simulink model "LW_ctrl_241029_1"  (R2024b)
settings: Solver=ode4  StartTime=0.0  StopTime=inf  FixedStep=0.005  RelTol=1e-3  EnableMultiTasking=on
StartFcn:
  | %timestart = cputime;
StopFcn:
  | %dt = cputime - timestart
undefined symbols (not defined in the file or in its folder): AttCtrl_cycle, ControlMode, DEG2RAD, Earth, FlightMode, LW_ACRO_P_MAX, LW_ACRO_R_MAX, LW_ACRO_Y_MAX, LW_AERO_C0, LW_AERO_C1, LW_AERO_Y0, LW_ANGLE, LW_DMZ0, LW_DMZ_MIN, LW_LAT_CIRCLE, LW_MAN_PITCH_MAX, LW_MAN_ROLL_MAX, LW_MASS, LW_OB_CIRCLE_R, LW_OB_CIRCLE_V, LW_OB_CIRCLE_W, LW_OB_TYPE, LW_REX_YAW, LW_SERVOL_MAX, LW_SERVOR_MAX, LW_TEST_DTXY, LW_TEST_DTZ, LW_THR_HOVER, LW_WZ_MAX, LW_X_ACCEL_MAX, LW_X_ACCEL_MIN, LW_X_FF, LW_X_JERK_MAX, LW_X_P, LW_X_VEL_MAX, LW_Y_ACCEL_MAX, LW_Y_ACCEL_MIN, LW_Y_FF, LW_Y_JERK_MAX, LW_Y_P, LW_Y_VEL_MAX, LW_YAW_KAD, LW_YAW_KAP, LW_Z_ACCEL_LOW, LW_Z_ACCEL_UP, LW_Z_FF, LW_Z_JERK_MAX, LW_Z_P, LW_Z_VEL_MAX_UP, Map_xoffset, Map_yoffset, Map_zoffset, MAX_wdotx, MAX_wdoty, MAX_wdotz, Mixer_cycle, ModelParam_AccelMax, ModelParam_DelayAtt, ModelParam_DelayOmega, ModelParam_DelayPos ... (+59)
libraries: pixhawk_slib_uORB_RW x15, simulink x7, slpidlib x6, dspfdesign x6, dspstat3 x5, aerolibnav x4, pixhawk_slib_sensors_actuators x3, aerolibtransform2 x3, etargetslib x2, pixhawk_slib_rfly x1, aerolibatmos2 x1, slrealtimeiplib x1
(part 5 of 6)

== matlab function LW_ctrl_241029_1/Controller/PID_Controller/PID_Controller/local_pos_ref_selector/position control ==
  data: manual_vel_ref input; manual_rates_ref input; offboard_ref input Bus: offboard_bus; timestamp input; vehicle_pos input; vehicle_vel input; delta_xy input size=2; xy_reset_counter input size=1; delta_z input size=1; z_reset_counter input size=1; delta_vxy input size=2; vxy_reset_counter input size=1; delta_vz input size=1; vz_reset_counter input size=1; delta_heading input size=1; heading_reset_counter input size=1; q input; wb input; states_flag input; dm_est input; ctrl_mode input; pos_ref output single; vd_lim output single; flight_mode input; arm input; yaw_ref output; wbz_ref output; man_acc_ff output; LW_WZ_MAX parameter; LW_X_P parameter; LW_Y_P parameter; LW_Z_P parameter; LW_LAT_CIRCLE parameter; LW_X_VEL_MAX parameter; LW_Z_VEL_MAX_UP parameter; LW_X_FF parameter size=1; LW_Y_FF parameter size=1; LW_Z_FF parameter size=1; LW_Y_ACCEL_MAX parameter; LW_REX_YAW parameter; LW_X_JERK_MAX parameter; LW_Y_JERK_MAX parameter; LW_Z_JERK_MAX parameter; LW_DMZ0 parameter; LW_DMZ_MIN parameter; LW_YAW_KAP parameter; LW_YAW_KAD parameter
function [pos_ref, vd_lim, yaw_ref, wbz_ref, man_acc_ff] = fcn(manual_vel_ref, manual_rates_ref, offboard_ref, ...
    timestamp, vehicle_pos, vehicle_vel, delta_xy, xy_reset_counter, delta_z, z_reset_counter,delta_vxy, vxy_reset_counter,delta_vz, vz_reset_counter,delta_heading, heading_reset_counter, q, wb, states_flag, dm_est, ctrl_mode, flight_mode, arm, ...
    LW_WZ_MAX, LW_X_P, LW_Y_P, LW_Z_P, LW_LAT_CIRCLE, LW_X_VEL_MAX, LW_Z_VEL_MAX_UP, LW_X_FF, LW_Y_FF, LW_Z_FF, LW_Y_ACCEL_MAX, LW_REX_YAW, LW_X_JERK_MAX, LW_Y_JERK_MAX, LW_Z_JERK_MAX,...
    LW_DMZ0, LW_DMZ_MIN, LW_YAW_KAP, LW_YAW_KAD)
%Function description:
%  Mode switch implementation.
%Input:
%  mode
%  manual_vel_ref：航向坐标系下的期望速度
%  vel_ref: The desired velocity specified by the remote control
%  x, y, z: current position
%  vx, vy,vz: current velocity
%Output:
%  pos_ref, vd_lim: desired velocity and position in NED

lw_acc_xy_max = LW_Y_ACCEL_MAX; %水平方向最大减速加速度
lw_acc_z_max = single(3.0);
if notInfNan(q)
    yaw = my_quat2yaw(q,'ZYX');%强制旋转次序，很有必要
else
    yaw = single(0);
end

%% persistent data define
persistent timestamp_last
if isempty(timestamp_last)
    timestamp_last = timestamp;
    dt = single(0.02);
else
    dt = single((timestamp - timestamp_last)*1e-6);
end
if dt > 0.2
    dt = single(0.2);
elseif dt < 0.001
    dt = single(0.001);
end
timestamp_last = timestamp;

persistent pos_x1 pos_y1 pos_z1
if isempty(pos_x1) || isempty(pos_y1) || isempty(pos_z1)
    if notInfNan(vehicle_pos)
        pos_x1 = vehicle_pos(1);
        pos_y1 = vehicle_pos(2);
        pos_z1 = vehicle_pos(3);
    else
        pos_x1 = single(0);
        pos_y1 = single(0);
        pos_z1 = single(0);
    end
end
persistent hold_xy_flag  hold_z_flag;
if isempty(hold_xy_flag) || isempty(hold_z_flag)
    hold_xy_flag = false;
    hold_z_flag = false;
end
persistent yaw_d_
if isempty(yaw_d_)
    if notInfNan(yaw)
        yaw_d_ = yaw;
    else
        yaw_d_ = single(0);
    end
end
persistent hold_xy_timestamp  hold_z_timestamp hold_vxy hold_pxy hold_vz hold_pz;
if isempty(hold_xy_timestamp) || isempty(hold_z_timestamp)
    hold_xy_timestamp = timestamp;
    hold_z_timestamp = timestamp;
end
if isempty(hold_vxy)
    hold_vxy = vehicle_vel(1:2);
end
if isempty(hold_pxy)
    hold_pxy = vehicle_pos(1:2);
end
if isempty(hold_pz)
    hold_pz = vehicle_pos(3);
end
if isempty(hold_vz)
    hold_vz = vehicle_vel(3);
end

persistent xy_reset_counter_ z_reset_counter_ vxy_reset_counter_ vz_reset_counter_ heading_reset_counter_
if isempty(heading_reset_counter_) || isempty(xy_reset_counter_) || isempty(z_reset_counter_) ...
        || isempty(vxy_reset_counter_) || isempty(vz_reset_counter_)
    xy_reset_counter_ = xy_reset_counter;
    z_reset_counter_ = z_reset_counter;
    vxy_reset_counter_ = vxy_reset_counter;
    vz_reset_counter_ = vz_reset_counter;
    heading_reset_counter_ = heading_reset_counter;
end

man_acc_ff = zeros(3,1,'single');
if notInfNan(flight_mode) && notInfNan(ctrl_mode) && arm == ControlMode.ARM
    %% yaw control
    relaxed_yaw = states_flag(1);
    wbz_ref = single(0);
    if flight_mode == FlightMode.PILOT && notInfNan(manual_rates_ref)...
            && ctrl_mode == ControlMode.POSITION
        if hold_xy_flag && LW_REX_YAW > 0.5 && abs(manual_rates_ref(3)) < 0.01
            Euler = my_quat2eul(q,'ZYX');
            dot_yaw = sin(Euler(1))/cos(Euler(2))*wb(2) + cos(Euler(1))/cos(Euler(2))*wb(3);
            if LW_YAW_KAD > 0.001
                [yaw_d_, dot_yaw_ref] = AdmittanceYaw(dm_est(3), yaw, dot_yaw, dt, LW_DMZ0, LW_DMZ_MIN, LW_YAW_KAP, LW_YAW_KAD, 0);
                wbz_ref = dot_yaw_ref*cos(Euler(1))*cos(Euler(2));
                wbz_ref = single(0);
            else
                roll_min = LW_DMZ_MIN;
                wv_gain = LW_YAW_KAP;
                roll_exceeding_treshold = single(0);
                if Euler(1) > roll_min
                    roll_exceeding_treshold = Euler(1) - roll_min;
                elseif Euler(1) < -roll_min
                    roll_exceeding_treshold = Euler(1) + roll_min;
                end
                yaw_d_ = yaw;
                wbz_ref = wv_gain*roll_exceeding_treshold;
            end
            %             if relaxed_yaw > 0.5
            %                 yaw_d_ = yaw;%悬停状态放宽偏航控制
            %             end
        else
            [~, ~] = AdmittanceYaw(dm_est(3), yaw, single(0), dt, LW_DMZ0, LW_DMZ_MIN, LW_YAW_KAP, LW_YAW_KAD, 1);%reset
            yaw_d_ = yaw_d_ + manual_rates_ref(3) * dt; %前飞状态允许手控偏航
        end
        if my_norm(vehicle_vel(1:2)) > 3 && abs(manual_vel_ref(2)) > 0.1
            yaw_d_ = yaw;
        end
    else
        yaw_d_ = yaw;
        [~, ~] = AdmittanceYaw(dm_est(3), yaw, single(0), dt, LW_DMZ0, LW_DMZ_MIN, LW_YAW_KAP, LW_YAW_KAD, 1); %reset
    end

    if flight_mode == FlightMode.PILOT
        %handle reset
        if heading_reset_counter_ ~= heading_reset_counter && abs(wrap_pi(yaw_d_ - yaw)) > 0.001
            yaw_d_ = yaw_d_ + delta_heading;
        end
        yaw_ref = yaw_d_;
    elseif flight_mode == FlightMode.OFFBOARD
        yaw_ref = my_quat2yaw(offboard_ref.q,'ZYX');%已经经过了reset补偿
    else
        yaw_ref = yaw_d_;
    end

    %限定偏航角的最大角度率
    LW_WZ_MAX_RAD = LW_WZ_MAX * pi / 180;
    %yaw_ref = limit_yaw(yaw_ref, dt, LW_WZ_MAX_RAD, arm);

    Rbe_psi = [ cos(yaw_d_) sin(yaw_d_) 0;
        -sin(yaw_d_) cos(yaw_d_) 0;
        0        0        1];

    %% select reference data
    if flight_mode == FlightMode.PILOT && (notInfNan(vehicle_pos) && notInfNan(vehicle_vel) && notInfNan(manual_vel_ref))
        vehicle_vel_psi = Rbe_psi*vehicle_vel;
        if ctrl_mode == ControlMode.STABILIZED || ctrl_mode == ControlMode.ACRO || ctrl_mode == ControlMode.MANUAL
            pos_x1 = vehicle_pos(1); pos_y1 = vehicle_pos(2); pos_z1 = vehicle_pos(3);
            hold_pxy = vehicle_pos(1:2); hold_pz = vehicle_pos(3);
            hold_vxy = vehicle_vel(1:2); hold_vz = vehicle_vel(3);
            hold_z_flag = false; hold_xy_flag = false;
            hold_xy_timestamp = timestamp; hold_z_timestamp = timestamp;
            vx_d = vehicle_vel_psi(1); vy_d = vehicle_vel_psi(2); vz_d = vehicle_vel_psi(3);
        elseif ctrl_mode == ControlMode.ALTITUDE
            pos_x1 = vehicle_pos(1); pos_y1 = vehicle_pos(2);
            hold_pxy = vehicle_pos(1:2);
            hold_vxy = vehicle_vel(1:2);
            hold_xy_flag = false;
            hold_xy_timestamp = timestamp;
            vx_d = vehicle_vel_psi(1); vy_d = vehicle_vel_psi(2);
            %判断是否需要定高
            if abs(manual_vel_ref(3)) < 0.001 && abs(vehicle_vel(3)) <= 0.8
                want_hold_z = true;
            else
                want_hold_z = false;
                hold_z_flag = false;
                hold_z_timestamp = timestamp;
                hold_vz = vehicle_vel(3);
                hold_pz = vehicle_pos(3);
            end

            if (want_hold_z) && (~hold_z_flag)
                %加入最大加速度限制
                time_to_stop = my_norm(hold_vz)/lw_acc_z_max;
                delta_t = single((timestamp - hold_z_timestamp)*1e-6);
                if delta_t > time_to_stop
                    delta_t = time_to_stop;
                    hold_z_flag = true;
                end
                pos_z1 = hold_pz + hold_vz*delta_t;
            end

            if ~want_hold_z
                pos_z1 = vehicle_pos(3);
                hold_z_flag = false;
            end
            vz_d = manual_vel_ref(3);
        else %position mode
            if abs(manual_vel_ref(1)) < 0.001 && abs(vehicle_vel_psi(1)) <= 0.8 && ...
                    abs(manual_vel_ref(2)) < 0.001 && abs(vehicle_vel_psi(2)) <= 0.8
                want_hold_xy = true;
            else
                want_hold_xy = false; hold_xy_flag = false;
                hold_xy_timestamp = timestamp;
                hold_vxy = vehicle_vel(1:2);
                hold_pxy = vehicle_pos(1:2);
            end
            if abs(manual_vel_ref(3)) < 0.001 && abs(vehicle_vel(3)) <= 0.8
                want_hold_z = true;
            else
                want_hold_z = false;
                hold_z_flag = false;
                hold_z_timestamp = timestamp;
                hold_vz = vehicle_vel(3);
                hold_pz = vehicle_pos(3);
            end

            vx_d = manual_vel_ref(1); vy_d = manual_vel_ref(2);
            vz_d = manual_vel_ref(3);
            %对手动期望速度进行平滑
            %             [vd_smoothed, ~] = TD_3DVector([vx_d;vy_d;vz_d], [lw_acc_xy_max;lw_acc_xy_max;lw_acc_z_max]*1.2, dt);
            %             vx_d = vd_smoothed(1);
            %             vy_d = vd_smoothed(2);
            %             vz_d = vd_smoothed(3);
            %让期望位置保持进入定点那刻的位置
            if (want_hold_xy) && (~hold_xy_flag)
                %加入最大加速度限制
                v0_xy = my_norm(hold_vxy(1:2));
                time_to_stop = v0_xy/lw_acc_xy_max;
                delta_t = single((timestamp - hold_xy_timestamp)*1e-6);
                if delta_t > time_to_stop
                    delta_t = time_to_stop;
                    hold_xy_flag = true;
                end

                pos_x1 = hold_pxy(1) + hold_vxy(1)*delta_t;
                pos_y1 = hold_pxy(2) + hold_vxy(2)*delta_t;

                %                 delta_vxy = v0_xy - lw_acc_xy_max*delta_t;
                %                 delta_pxy = v0_xy*delta_t - 0.5*lw_acc_xy_max*delta_t^2;
                %                 pos_x1 = hold_pxy(1) + delta_pxy*cos(yaw_d_);
                %                 pos_y1 = hold_pxy(2) + delta_pxy*sin(yaw_d_);

                %直接停住
                %                     x1 = vehicle_pos(1); y1 = vehicle_pos(2);
                %                     hold_xy_flag = true;
            end

            % throttle in the middle position, hold the height
            if (want_hold_z) && (~hold_z_flag)
                %加入最大加速度限制
                time_to_stop = my_norm(hold_vz)/lw_acc_z_max;
                delta_t = single((timestamp - hold_xy_timestamp)*1e-6);
                if delta_t > time_to_stop
                    delta_t = time_to_stop;
                    hold_z_flag = true;
                end
                pos_z1 = hold_pz + hold_vz*delta_t;
            end
            %When the RC sticks(CH1, CH2, CH3, CH4) deviate from the middle dead zone range, the position is the current position.
            %The position controller only works with the velocity loop
            if ~want_hold_xy
                pos_x1 = vehicle_pos(1); pos_y1 = vehicle_pos(2);
                hold_xy_flag = false;
            end
            if ~want_hold_z
                pos_z1 = vehicle_pos(3); hold_z_flag = false;
            end

        end
        vel_ref = [vx_d; vy_d; vz_d]; %航向坐标系下的期望速度
        pos_ref = [pos_x1; pos_y1; pos_z1];

        % 状态reset处理
        delta_v = Rbe_psi *[delta_vxy;delta_vz];
        if vxy_reset_counter_ ~= vxy_reset_counter && my_norm(vel_ref(1:2) - vehicle_vel(1:2)) > 0.001
            vel_ref(1:2) = vel_ref(1:2) + delta_v(1:2);
        end
        if vz_reset_counter_ ~= vz_reset_counter && abs(vel_ref(3) - vehicle_vel(3)) > 0.001
            vel_ref(3) = vel_ref(3) +  delta_v(3);
        end
        if xy_reset_counter_ ~= xy_reset_counter && my_norm(pos_ref(1:2) - vehicle_pos(1:2)) > 0.001
            pos_ref(1:2) = pos_ref(1:2) + delta_xy;
            pos_x1 = pos_ref(1);
            pos_y1 = pos_ref(2);
        end
        if z_reset_counter_ ~= z_reset_counter && abs(pos_ref(3) - vehicle_pos(3)) > 0.001
            pos_ref(3) = pos_ref(3) + delta_z;
            pos_z1 = pos_ref(3);
        end
        xy_reset_counter_ = xy_reset_counter;
        z_reset_counter_ = z_reset_counter;
        vxy_reset_counter_ = vxy_reset_counter;
        vz_reset_counter_ = vz_reset_counter;
        heading_reset_counter_ = heading_reset_counter;
        %
        %     elseif flight_mode == FlightMode.AUTO && notInfNan(vehicle_pos) % auto
        %         dubins = auto_ref.dubins;
        %         pos_ref = [vehicle_pos(1 : 2); -non_manual_ref.current.alt];
        %         vel_ref = [non_manual_ref.current.cruising_speed; 0; 0];
        %         x1 = vehicle_pos(1); y1 = vehicle_pos(2); z1 = vehicle_pos(3);
        %         if ctrl_mode == ControlMode.LOITER && (notInfNan(non_manual_ref.current.pos) && notInfNan(non_manual_ref.current.vel))
        %             pos_ref = non_manual_ref.current.pos;
        %             vel_ref = non_manual_ref.current.vel;
        %         end
    elseif flight_mode == FlightMode.OFFBOARD && (notInfNan(vehicle_pos)) % offboard
        if notInfNan(offboard_ref.pos)
            pos_ref = offboard_ref.pos;
        else
            pos_ref = vehicle_pos;
        end
        if notInfNan(offboard_ref.vel)
            vel_ref = offboard_ref.vel;
        else
            vel_ref = zeros(3,1,'single');
        end

        pos_x1 = vehicle_pos(1); pos_y1 = vehicle_pos(2); pos_z1 = vehicle_pos(3);
        hold_pxy = vehicle_pos(1:2); hold_pz = vehicle_pos(3);
        hold_vxy = vehicle_vel(1:2); hold_vz = vehicle_vel(3);
        hold_z_flag = false; hold_xy_flag = false;
        hold_xy_timestamp = timestamp; hold_z_timestamp = timestamp;
    else
        vel_ref = single([0; 0; 0]);
        pos_ref = [pos_x1; pos_y1; pos_z1];
    end


    %% position control
    vel_fb = (pos_ref - vehicle_pos).* [LW_X_P; LW_Y_P; LW_Z_P];
    vd_psi = Rbe_psi *vel_fb + vel_ref; %手控模式下参考速度vel_ref是航向坐标系下的
    if flight_mode == FlightMode.AUTO  %not used, replaced by the L1 in PX4
        if vel_ref(2) < 1e-3
            vd_psi(2) = vel_fb(2);
        else
            %对圆轨迹跟踪，d为半径误差
            vd_psi(2) = single(LW_LAT_CIRCLE * vel_ref(2));
        end
    end

    vd_lim = Rbe_psi'*vd_psi;%将期望速度转换到NED下
    if (flight_mode == FlightMode.PILOT && (ctrl_mode == ControlMode.ALTITUDE || ctrl_mode == ControlMode.POSITION )) ...
            || flight_mode == FlightMode.AUTO
        %z-axis保大小
        vd_psi(3) = constrain(vd_psi(3), -LW_Z_VEL_MAX_UP, LW_Z_VEL_MAX_UP);

        if (flight_mode == FlightMode.PILOT && (ctrl_mode == ControlMode.POSITION )) || flight_mode == FlightMode.AUTO
            %xy-axis保方向
            vd_xy_norm = sqrt(vd_psi(1) * vd_psi(1) + vd_psi(2) * vd_psi(2));
            VEL_MAX_XY = LW_X_VEL_MAX;
            if vd_xy_norm > VEL_MAX_XY
                vd_psi(1 : 2) = vd_psi(1 : 2) * VEL_MAX_XY / vd_xy_norm;
            end
        end
        [vd_psi, man_acc_ff] = TD_3DVector(vd_psi, ([LW_X_JERK_MAX; LW_Y_JERK_MAX; LW_Z_JERK_MAX]), dt);
        man_acc_ff = zeros(3,1,'single');%手动控制加速度前馈
        vd_lim = Rbe_psi'*vd_psi;
    end
    if flight_mode == FlightMode.OFFBOARD
        vel_fb = ((pos_ref - vehicle_pos)).* [LW_X_P; LW_Y_P; LW_Z_P];
        vd_lim = vel_fb + vel_ref.* [LW_X_FF; LW_Y_FF; LW_Z_FF];
    end
else
    if notInfNan(vehicle_pos)
        pos_ref = vehicle_pos;
    else
        pos_ref = single([0; 0; 0]);
    end
    vd_lim = single([0; 0; 0]);
    yaw_ref = yaw;
    wbz_ref = single(0);
    [~, ~] = AdmittanceYaw(dm_est(3), yaw, single(0), dt, LW_DMZ0, LW_DMZ_MIN, LW_YAW_KAP, LW_YAW_KAD, 1); %reset

    pos_x1 = vehicle_pos(1); pos_y1 = vehicle_pos(2); pos_z1 = vehicle_pos(3);
    hold_pxy = vehicle_pos(1:2); hold_pz = vehicle_pos(3);
    hold_vxy = vehicle_vel(1:2); hold_vz = vehicle_vel(3);
    hold_z_flag = false; hold_xy_flag = false;
    hold_xy_timestamp = timestamp; hold_z_timestamp = timestamp;
    yaw_d_ = yaw;

    xy_reset_counter_ = xy_reset_counter;
    z_reset_counter_ = z_reset_counter;
    vxy_reset_counter_ = vxy_reset_counter;
    vz_reset_counter_ = vz_reset_counter;
    heading_reset_counter_ = heading_reset_counter;
end
%yaw_ref = my_quat2yaw(offboard_ref.q,'ZYX');
%yaw_ref = single(45/180*pi);
end

function [yaw_ref, dot_yaw_ref] = AdmittanceYaw(dmz, yaw, dot_yaw, dt, dmz0, dmz_min, k_ap, k_ad, reset)
% 偏航导纳控制
% 误差形式：
% e = yaw_ref - yaw
% k_ap*e + k_ad*dote = dmz
% 输入：
% dmz         - 估计偏航力矩扰动 d_m_est_z
% yaw         - 偏航角 \psi
% dot_yaw     - 偏航导数 \dot{\psi}
% dt          - 采样时间间隔
% 输出：
% yaw_ref     - 期望偏航角
% dot_yaw_ref - 期望偏航角速率
% 参数：
% k_ad        - 调节参数 k_{\text{ad}}
% k_ap        - 调节参数 k_{\text{ap}}


persistent yawerror_last yaw_ref_last
if isempty(yawerror_last) || isempty(yaw_ref_last)
    yawerror_last = single(0);
    yaw_ref_last =  yaw;
end

% k_ap = 1; k_ad = 1.0;
% dmz0 = -0.023;
if reset > 0.5
    yawerror_last = single(0);
    yaw_ref_last =  yaw;
    yaw_ref = yaw;
    dot_yaw_ref = single(0);
else
    dmz = dmz - dmz0;
    if abs(dmz) <= dmz_min
        dmz = single(0);
    end
    dot_yaw_ref = dot_yaw + 1/k_ad*(-k_ap*yawerror_last + dmz);
    yawerror_last = yawerror_last + (dot_yaw_ref - dot_yaw)*dt;
    yaw_ref = yaw + yawerror_last;

    if abs(dmz) <= dmz_min
        yaw_ref = yaw_ref_last;
    else
        yaw_ref_last = yaw_ref;
    end
end

end

function yaw_lim = limit_yaw(yaw_ref, dt, wz_max, arm)
persistent yaw_d_last;
if isempty(yaw_d_last)
    yaw_d_last = single(yaw_ref);
end
yaw_error = yaw_ref - yaw_d_last;
yaw_error = wrap_pi(yaw_error);
yawrate_ref = yaw_error / dt;

if yawrate_ref > wz_max
    yaw_ref = yaw_d_last + wz_max * dt;
elseif yawrate_ref < -wz_max
    yaw_ref = yaw_d_last - wz_max * dt;
end
yaw_lim = wrap_pi(yaw_ref);
if arm == ControlMode.ARM
    yaw_d_last = yaw_lim;
else
    yaw_d_last = yaw_ref;
end
end

function [v1_, v2_] = TD_3DVector(v, r, h)
%v:[3,1]
%r:[3,1]
%h:1
persistent v1 v2
if isempty(v1) || isempty(v2)
    v1 = single([0;0;0]);
    v2 = single([0;0;0]);
end
v = single(v);
r = single(r);
h = single(h);

v1_ = v1;
v2_ = v2;
for i = 1:3
    fv = fhan(v1(i) - v(i), v2(i), r(i),  h);
    v1_(i) = v1(i) + h*v2(i);
    v2_(i) = v2(i) + h*fv;
end

if notInfNan(v1_) && notInfNan(v2_)
    v1 = v1_;
    v2 = v2_;
end
end

function y = fhan(x1, x2, r0, h0)

d = r0*h0^2;
a0 = h0*x2;
y = x1 + a0;
a1 = sqrt(d*(d + 8*abs(y)));
a2 = a0 + sign(y)*(a1 - d)/2;
sy = (sign(y + d) - sign(y - d))/2;%fsg
a = (a0 + y -a2)*sy + a2;
sa = (sign(a + d) - sign(a - d))/2;
y = -r0*(a/d - sign(a))*sa - r0*sign(a);

end

== matlab function LW_ctrl_241029_1/navigator/navigator_manual/nan_inf11 ==
  data: u input; y output
function y = fcn(u)

for i = 1:length(u)
    if isnan(u(i)) || isinf(u(i))
        u(i) = single(0);
    end
end
y = u;

== matlab function LW_ctrl_241029_1/navigator/navigator_manual/nan_inf9 ==
  data: u input; y output
function y = fcn(u)

for i = 1:length(u)
    if isnan(u(i)) || isinf(u(i))
        u(i) = single(0);
    end
end
y = u;

== matlab function LW_ctrl_241029_1/navigator/navigator_manual/pitchrate_deadzone1 ==
  data: u input; y output
function y = fcn(u)
%Function description:
%  set a dead zone with a dead zone size of ±deadZone.
RCMin = single(-1);
RCMax = single(1);
RCMid = ((RCMin + RCMax)/2);
deadZone = 0;
k = 1/(RCMax - RCMid - deadZone);

%dead zone
if(u > RCMid + deadZone)
    y = single((u-RCMid - deadZone)*k);
elseif(u < RCMid - deadZone)
    y = single((u - RCMid + deadZone)*k);
else
    y = single(0);
end
end

== matlab function LW_ctrl_241029_1/Controller/PID_Controller/PID_Controller/altitude control/attrates_ref_selector ==
  data: flight_mode input; arm input; ctrl_mode input; rate_ctrl_integral_reset output
function rate_ctrl_integral_reset = fcn(flight_mode, arm, ctrl_mode)

rate_ctrl_integral_reset = [true; true; true];
if notInfNan(flight_mode) && notInfNan([ctrl_mode, arm])
    if  arm == ControlMode.DISARM || ctrl_mode == ControlMode.MANUAL
        rate_ctrl_integral_reset = [true; true; true];
    else
        rate_ctrl_integral_reset = [false; false; false];
    end
end

end

== matlab function LW_ctrl_241029_1/Controller/PID_Controller/PID_Controller/postion control/nan_inf_mode ==
  data: u input; y output
function y = fcn(u)

for i = 1:length(u)
    if isnan(u(i)) || isinf(u(i))
        u(i) = ControlMode.DISARM;
    end
end
y = u;

== matlab function LW_ctrl_241029_1/Controller/PID_Controller/PID_Controller/postion control/pos_ctrl_integral_reset ==
  data: ctrl_mode input; integral_reset output boolean
function integral_reset = fcn(ctrl_mode)
mode = ctrl_mode(1);
arm = ctrl_mode(2);
if mode == ControlMode.ACRO || mode == ControlMode.STABILIZED || mode == ControlMode.MANUAL || arm == ControlMode.DISARM
    integral_reset = [true true];
elseif mode == ControlMode.ALTITUDE
    integral_reset = [true false];
elseif mode == ControlMode.POSITION
    integral_reset = [false false];
else
    integral_reset = [false false];
end

== matlab function LW_ctrl_241029_1/Controller/PID_Controller/PID_Controller/postion control/pos_ctrl_integral_reset2 ==
  data: v_ned input; v_body output; psi input
function v_body = fcn(v_ned, psi)
    % 构造旋转矩阵
    R = [cos(psi), sin(psi), 0;
         -sin(psi), cos(psi), 0;
         0, 0, 1];

    % 转换速度
    v_body = R * [v_ned(1);v_ned(2);v_ned(3)];
end

== matlab function LW_ctrl_241029_1/Controller/PID_Controller/PID_Controller/postion control/pos_ctrl_integral_reset3 ==
  data: eax input; phi_d output; eay input; theta_d output
function [phi_d,theta_d] = fcn(eax,eay)

g = 9.8;
phi_d = atan(eay/g);
theta_d = -atan(eax/g);

== matlab function LW_ctrl_241029_1/Controller/PID_Controller/PID_Controller/select parameter/MATLAB Function ==
  data: u input; y output
function y = fcn(u)

y = my_quat2eul(u);

== matlab function LW_ctrl_241029_1/Controller/PID_Controller/PID_Controller/altitude control/MATLAB Function ==
  data: f_d input; Mx_d input; My_d input; T1 output; Mz_d input; T2 output; T3 output; T4 output; ModelParam_uavJ parameter
function [T1,T2,T3,T4] = fcn(f_d,Mx_d,My_d,Mz_d,ModelParam_uavJ)


u = ModelParam_uavJ*[Mx_d;My_d;Mz_d];
fM_d = [f_d;u];
Allocation = [0.2500   -1.1765    1.0000   15.0602
    0.2500   -1.1765   -1.0000  -15.0602
    0.2500    1.1765    1.0000  -15.0602
    0.2500    1.1765   -1.0000   15.0602];

T = Allocation*fM_d;
if T(1)<0
    T1 = single(0);
else
    T1 = T(1);
end
if T(2)<0
    T2 = single(0);
else
    T2 = T(2);
end
if T(3)<0
    T3 = single(0);
else
    T3 = T(3);
end
if T(4)<0
    T4 = single(0);
else
    T4 = T(4);
end

== matlab function LW_ctrl_241029_1/Controller/PID_Controller/PID_Controller/altitude control/MATLAB Function1 ==
  data: quat input; euler_d input; psi_err output; phi_err output; theta_err output
function [psi_err,phi_err,theta_err] = fcn(quat,euler_d)

quat_d = my_eul2quat(euler_d);
euler = my_quat2eul(quat);

% quat_d, quat: 1x4, [w x y z]
q_err = quatmultiply(quat_d', quatinv(quat')); 

eul_err = quat2eul(q_err, "ZYX");              
psi_err = 3*wrapToPi(eul_err(1));                
phi_err = 10*(euler_d(1) - euler(1));
theta_err = 10*(euler_d(2) - euler(2));

== matlab function LW_ctrl_241029_1/Controller/PID_Controller/PID_Controller/postion control/pos_ctrl_integral_reset1 ==
  data: v_ned input; psi input; v_body output
function v_body  = fcn(v_ned, psi)
    % 构造旋转矩阵
    R = [cos(psi), sin(psi), 0;
         -sin(psi), cos(psi), 0;
         0, 0, 1];

    % 转换速度
    v_body = R * [v_ned(1);v_ned(2);v_ned(3)];
end

== matlab function LW_ctrl_241029_1/navigator/navigator_manual/rollrate_deadzone1 ==
  data: u input; y output
function y = fcn(u)
%Function description:
%  set a dead zone with a dead zone size of ±deadZone.
RCMin = single(-1);
RCMax = single(1);
RCMid = ((RCMin + RCMax)/2);
deadZone = 0;
k = 1/(RCMax - RCMid - deadZone);

%dead zone
if(u > RCMid + deadZone)
    y = single((u-RCMid - deadZone)*k);
elseif(u < RCMid - deadZone)
    y = single((u - RCMid + deadZone)*k);
else
    y = single(0);
end
end

== matlab function LW_ctrl_241029_1/navigator/navigator_manual/yawrate_deadzone1 ==
  data: u input; y output
function y = fcn(u)
%Function description:
%  set a dead zone with a dead zone size of ±deadZone.
RCMin = single(-1);
RCMax = single(1);
RCMid = ((RCMin + RCMax)/2);
deadZone = 0;
k = 1/(RCMax - RCMid - deadZone);

%dead zone
if(u > RCMid + deadZone)
    y = single((u-RCMid - deadZone)*k);
elseif(u < RCMid - deadZone)
    y = single((u - RCMid + deadZone)*k);
else
    y = single(0);
end
end

== matlab function LW_ctrl_241029_1/rc_receive/manual_ctrl_in/Sim/Simulate ref/commandMapping/command2pwm/man/delta_e_inv ==
  data: u input; y output
function y = fcn(u)
%Function description:
%  set a dead zone with a dead zone size of ±deadZone.
RCMin = single(-1);
RCMax = single(1);
RCMid = ((RCMin + RCMax)/2);
deadZone = 0;
k = 1/(RCMax - RCMid - deadZone);

%dead zone
if(u > RCMid + deadZone)
    y = single(u/k + RCMid + deadZone);
elseif(u < RCMid - deadZone)
     y = single(u/k + RCMid - deadZone);
else
    y = single(0);
end
end

== matlab function LW_ctrl_241029_1/rc_receive/manual_ctrl_in/Sim/Simulate ref/commandMapping/command2pwm/man/delta_a_inv ==
  data: u input; y output
function y = fcn(u)
%Function description:
%  set a dead zone with a dead zone size of ±deadZone.
RCMin = single(-1);
RCMax = single(1);
RCMid = ((RCMin + RCMax)/2);
deadZone = 0;
k = 1/(RCMax - RCMid - deadZone);

%dead zone
if(u > RCMid + deadZone)
    y = single(u/k + RCMid + deadZone);
elseif(u < RCMid - deadZone)
     y = single(u/k + RCMid - deadZone);
else
    y = single(0);
end
end

== matlab function LW_ctrl_241029_1/rc_receive/manual_ctrl_in/Sim/Simulate ref/commandMapping/command2pwm/man/delta_r_inv ==
  data: u input; y output
function y = fcn(u)
%Function description:
%  set a dead zone with a dead zone size of ±deadZone.
RCMin = single(-1);
RCMax = single(1);
RCMid = ((RCMin + RCMax)/2);
deadZone = 0;
k = 1/(RCMax - RCMid - deadZone);

%dead zone
if(u > RCMid + deadZone)
    y = single(u/k + RCMid + deadZone);
elseif(u < RCMid - deadZone)
     y = single(u/k + RCMid - deadZone);
else
    y = single(0);
end
end

== matlab function LW_ctrl_241029_1/states_update/vehicle_local_position/Sim/nan_inf ==
  data: u input; y output
function y = fcn(u)

for i = 1:length(u)
    if isnan(u(i)) || isinf(u(i))
        u(i) = single(0);
    end
end
y = u;

== matlab function LW_ctrl_241029_1/states_update/vehicle_local_position/Sim/nan_inf1 ==
  data: u input; y output
function y = fcn(u)

for i = 1:length(u)
    if isnan(u(i)) || isinf(u(i))
        u(i) = single(0);
    end
end
y = u;

== stateflow chart LW_ctrl_241029_1/Scheduler ==
  state Scheduler
    on every(StatesUpdate_cycle,tick):send(StatesUpdate);
    on every(AttCtrl_cycle,tick):send(AttCtrl);
    on every(Mixer_cycle,tick):send(Mixer);
    on every(PosCtrl_cycle,tick):send(PosCtrl);
    on every(Navigator_cycle,tick):send(Navigator);
    on every(StateMachine_cycle,tick):send(StateMachine);
    on every(RCReceive_cycle,tick):send(RCReceive);
  (default) -> Scheduler
  data: AttCtrl_cycle parameter; Mixer_cycle parameter; StateMachine_cycle parameter; PosCtrl_cycle parameter; Navigator_cycle parameter; RCReceive_cycle parameter; StatesUpdate_cycle parameter
  events: Mixer output FUNCTION_CALL_EVENT; AttCtrl output FUNCTION_CALL_EVENT; PosCtrl output FUNCTION_CALL_EVENT; Navigator output FUNCTION_CALL_EVENT; StateMachine output FUNCTION_CALL_EVENT; RCReceive output FUNCTION_CALL_EVENT; StatesUpdate output FUNCTION_CALL_EVENT

== matlab function LW_ctrl_241029_1/Output/OutputSelect/Sim/Lifting Body Airframe/Estimator/GPS/courseAngle ==
  data: v input; course_angle output; euler input
function course_angle = fcn(v, euler)

if norm(v) < 0.1
    course_angle = euler(3);
else
    course_angle = atan2(v(2),v(1));
end

== matlab function LW_ctrl_241029_1/rc_receive/manual_ctrl_in/Sim/joystick/MATLAB Function1 ==
  data: x output; ch1 input; y output; ch2 input; ch3 input; ch4 input; states input; failsafe input; rc_lost input; RC1_MIN parameter single size=1; RC1_MAX parameter single size=1; RC1_REV parameter single size=1; RC2_MIN parameter single size=1; RC2_MAX parameter single size=1; RC2_REV parameter single size=1; RC3_MIN parameter single size=1; RC3_MAX parameter single size=1; RC3_REV parameter single size=1; RC4_MIN parameter single size=1; RC4_MAX parameter single size=1; RC4_REV parameter single size=1; z output; r output; AU5 output; AU6 output; AU7 output; AU8 output; RC_LOST output
function [x, y, z, r, AU5, AU6, AU7, AU8, RC_LOST] = fcn(ch1, ch2, ch3, ch4, states, failsafe, rc_lost, ...
    RC1_MIN, RC1_MAX, RC1_REV, RC2_MIN, RC2_MAX, RC2_REV, RC3_MIN, RC3_MAX, RC3_REV, RC4_MIN, RC4_MAX, RC4_REV)

persistent rc_lost_count
if isempty(rc_lost_count)
    rc_lost_count = single(0.0);
end

x = rcNormalize(single(ch2), RC2_MIN, RC2_MAX, RC2_REV, single(0.0));
x = constrain(x, single(-1), single(1));
y = rcNormalize(single(ch1), RC1_MIN, RC1_MAX, RC1_REV, single(0.0));
y = constrain(y, single(-1), single(1));
z = rcNormalize(single(ch3), RC3_MIN, RC3_MAX, RC3_REV, single(0.0));
z = constrain(z, single(-1), single(1));
r = rcNormalize(single(ch4), RC4_MIN, RC4_MAX, RC4_REV, single(0.0));
r = constrain(r, single(-1), single(1));
%ch5:[0,1]
%ch6:[0,2];
%ch7:[0,4];
%ch8:[0,8]
%arm:0;disarm>=1
%stabilize:1;altitude:2;position:3;
%
AU5 = single(1000);
AU6 = single(1000);
AU7 = single(1000);
AU8 = single(1000);
if states >= 1
    AU6 = single(2000);
    switch states
        case 1 % stabilize
            AU5 = single(1000);
            AU7 = single(1000);
            AU8 = single(1000);
        case 2 % altitude
            AU5 = single(1500);
            AU7 = single(1000);
            AU8 = single(1000);
        case 3 % position
            AU5 = single(2000);
            AU7 = single(1000);
            AU8 = single(1000);
        otherwise
            AU5 = single(1000);
            AU7 = single(1000);
            AU8 = single(1000);
    end
end

RC_LOST = single(0.0);
if rc_lost > single(0.5) || failsafe > single(0.5)
    rc_lost_count = rc_lost_count + single(1);
    if rc_lost_count > single(5)
        RC_LOST = single(1.0);
        rc_lost_count = single(5);
    end
else
    rc_lost_count = single(0.0);
end

== matlab function LW_ctrl_241029_1/Output/OutputSelect/Sim/Lifting Body Airframe/Estimator/Sensor Model/GPS/-pi-pi---->0-2pi ==
  data: yaw180 input; yaw360 output
function yaw360 = fcn(yaw180)
%//rad
if yaw180>0
    yaw360 = yaw180;
else
    yaw360 = yaw180 +2*pi;
end

== matlab function LW_ctrl_241029_1/states_update/vehicle_local_position/HIL&FLY V1.13.3/getIncid ==
  data: q input; incid output; LW_ANGLE parameter
function incid = fcn(q, LW_ANGLE)

if notInfNan(q)
    euler = my_quat2eul(q);
else
    euler = single([0;0;0]);
end
theta = euler(2);
alpha = theta + LW_ANGLE*pi/180;
beta = single(0);
incid = [alpha; beta];

== matlab function LW_ctrl_241029_1/state_machine/MATLAB Function3 ==
  data: ch6 input; arm output; armed input
function arm  = fcn(ch6, armed)
%Function description:
%  the remote control CH6 channel arm or disarm the vehicle
%input:
%  ch6: Remote control CH6 channel input

% if ch6 > 1700 || armed == 1
%     arm = ControlMode.ARM;
% else
%     arm = ControlMode.DISARM;
% end

if ch6 < 1700 && armed == 0
    arm = ControlMode.DISARM;
else
    arm = ControlMode.ARM;
end

== matlab function LW_ctrl_241029_1/states_update/vehicle_local_position/HIL&FLY V1.13.3/nan_inf ==
  data: u input; y output
function y = fcn(u)

for i = 1:length(u)
    if isnan(u(i)) || isinf(u(i))
        u(i) = single(0);
    end
end
y = u;

== matlab function LW_ctrl_241029_1/rc_receive/manual_ctrl_in/Sim/Simulate RC/InputConditioning/deadzone0 ==
  data: u input; y output; rc_min input; rc_max input
function y = fcn(u, rc_min, rc_max)
%Function description:
%  Control the range of the remote control input from RCMin to RCMax, and set
%  a dead zone with a dead zone size of ±deadZone,the output y is
%  normalized to 0~1.You can get the RC calibration parameters in QGC.
RCMin = rc_min;
RCMax = rc_max;
RCMid = ((RCMin + RCMax)/2);
deadZoneRate = double(0.05);
deadZone = deadZoneRate*(RCMax - RCMin);
k = 1/(RCMax - RCMid - deadZone);
%Limiting
if(u < RCMin)
    u = RCMin;
elseif(u > RCMax)
    u = RCMax;
end
%dead zone and normalize
 if(u > RCMid + deadZone)
    y = single((u-RCMid - deadZone)*k);
 elseif(u < RCMid - deadZone)
     y = single((u - RCMid + deadZone)*k);
 else
     y = single(0);
 end
 end

== matlab function LW_ctrl_241029_1/states_update/vehicle_local_position/HIL&FLY V1.13.3/nan_inf_q ==
  data: u input; y output
function y = fcn(u)

for i = 1:length(u)
    if isnan(u(i)) || isinf(u(i))
        if i == 1
            u(i) = single(1);
        else
            u(i) = single(0);
        end
    end
end
y = u;

== matlab function LW_ctrl_241029_1/rc_receive/manual_ctrl_in/HIL&FLY V1.13.3/MATLAB Function ==
  data: x output; ch1 input; y output; ch2 input; ch3 input; ch4 input; ch5 input; ch6 input; ch7 input; ch8 input; failsafe input; rc_lost input; RC1_MIN parameter single size=1; RC1_MAX parameter single size=1; RC1_REV parameter single size=1; RC2_MIN parameter single size=1; RC2_MAX parameter single size=1; RC2_REV parameter single size=1; RC3_MIN parameter single size=1; RC3_MAX parameter single size=1; RC3_REV parameter single size=1; RC4_MIN parameter single size=1; RC4_MAX parameter single size=1; RC4_REV parameter single size=1; z output; r output; AU5 output; AU6 output; AU7 output; AU8 output; RC_LOST output
function [x, y, z, r, AU5, AU6, AU7, AU8, RC_LOST] = fcn(ch1, ch2, ch3, ch4, ch5, ch6, ch7, ch8, failsafe, rc_lost,...
RC1_MIN, RC1_MAX, RC1_REV, RC2_MIN, RC2_MAX, RC2_REV, RC3_MIN, RC3_MAX, RC3_REV, RC4_MIN, RC4_MAX, RC4_REV)

persistent rc_lost_count
if isempty(rc_lost_count)
   rc_lost_count = single(0.0); 
end
x = rcNormalize(single(ch2), RC2_MIN, RC2_MAX, RC2_REV,single(0.0));
x = constrain(x, single(-1), single(1));
y = rcNormalize(single(ch1), RC1_MIN, RC1_MAX, RC1_REV,single(0.0));
y = constrain(y, single(-1), single(1));
z = rcNormalize(single(ch3), RC3_MIN, RC3_MAX, RC3_REV,single(0.0));
z = (z + 1)*0.5;
z = constrain(z, single(0), single(1));
r = rcNormalize(single(ch4), RC4_MIN, RC4_MAX, RC4_REV,single(0.0));
r = constrain(r, single(-1), single(1));
AU5 = single(ch5);
AU6 = single(ch6);
AU7 = single(ch7);
AU8 = single(ch8);
RC_LOST = single(0.0);
if rc_lost > single(0.5) || failsafe > single(0.5)
    rc_lost_count = rc_lost_count + single(1);
    if rc_lost_count > single(5)
        RC_LOST = single(1.0);
        rc_lost_count = single(5);
    end
else
   rc_lost_count = single(0.0); 
end

== matlab function LW_ctrl_241029_1/states_update/vehicle_local_position/HIL&FLY V1.13.3/LW_LED ==
  data: y output; LW_LED parameter
function y = fcn(LW_LED)

y = [LW_LED 0 0];

== matlab function LW_ctrl_241029_1/Output/OutputSelect/Sim/Lifting Body Airframe/Estimator/nan_inf7 ==
  settings: updateMethod=DISCRETE
  data: timestamp input; delta_xy output; xy_reset_counter output; delta_z output; z_reset_counter output; delta_vxy output; vxy_reset_counter output; delta_vz output; vz_reset_counter output; heading output; delta_heading output; heading_reset_counter output; p input; v input; q input; ModelReset_time parameter; delta_q_reset output; quat_reset_counter output; ModelReset_Euler parameter; ModelReset_Pos parameter
function [delta_xy, xy_reset_counter, delta_z, z_reset_counter, delta_vxy,vxy_reset_counter,delta_vz, vz_reset_counter,heading, delta_heading, heading_reset_counter, delta_q_reset, quat_reset_counter]  = fcn(timestamp,p,v,q,ModelReset_time,ModelReset_Euler, ModelReset_Pos)

 persistent p_last v_last heading_last q_last
% persistent xy_reset_counter_  z_reset_counter_   vxy_reset_counter_  vz_reset_counter_ heading_reset_counter_
if isempty(p_last)
    p_last = p;
    v_last = v;
    heading_last = quat2yaw(q);
    q_last = q;
end
% 
% if isempty(xy_reset_counter_)
%     xy_reset_counter_ = single(0);
%     z_reset_counter_ = single(0);
%     vxy_reset_counter_ = single(0);
%     vz_reset_counter_ = single(0);
%     heading_reset_counter_ = single(0);
% end
% persistent resetNum delta_xy_  delta_z_ delta_vxy_  delta_vz_ delta_heading_ delta_q_reset_
% if isempty(resetNum)
%     resetNum = single(1);
%     delta_xy_ = single([0;0]);
%     delta_z_ = single(0);
%     delta_vxy_ = single([0;0]);
%     delta_vz_ = single(0);
%     delta_heading_ = single(0);
%     delta_q_reset_ = single([1;0;0;0]);
% end
% 
heading = quat2yaw(q);
% 
% if resetNum <= length(ModelReset_time)
%     if timestamp >= ModelReset_time(resetNum)
%         
% %         delta_p = p - p_last;
%          delta_v = v - v_last;
% %         delta_xy_ = delta_p(1:2);
% %         delta_z_ = delta_p(3);
% %         delta_vxy_= delta_v(1:2);
% %         delta_vz_ = delta_v(3);
% %         delta_heading_ = heading - heading_last;
% %         delta_q = quatmultiply(q(:)',quatconj(q_last(:)'));
% %         delta_q_reset_ = delta_q(:);
%         delta_xy_ = single(ModelReset_Pos(resetNum,1:2)');
%         delta_z_ = single(ModelReset_Pos(resetNum,3));
%         delta_vxy_= delta_v(1:2);
%         delta_vz_ = delta_v(3);
%         delta_heading_ = single(ModelReset_Euler(resetNum,3));
%         delta_q = eul2quat([ModelReset_Euler(resetNum,3) ModelReset_Euler(resetNum,2) ModelReset_Euler(resetNum,1)],'ZYX');
%         delta_q_reset_ = single(delta_q(:));
%         resetNum = resetNum + 1;
%     else
%         p_last = p;
%         v_last = v;
%         heading_last = heading;
%     end
% else
%     p_last = p;
%     v_last = v;
%     heading_last = heading;
% end
% delta_xy = delta_xy_;
% delta_z = delta_z_;
% delta_vxy = delta_vxy_;
% delta_vz = delta_vz_;
% delta_heading = delta_heading_;
% delta_q_reset = delta_q_reset_;
% 
% xy_reset_counter = resetNum - 1;
% z_reset_counter = resetNum - 1;
% vxy_reset_counter = resetNum - 1;
% vz_reset_counter = resetNum - 1;
% heading_reset_counter = resetNum - 1;
% quat_reset_counter = resetNum - 1;

persistent    delta_v_  v_reset_counter_
if isempty(delta_v_) || isempty(v_reset_counter_)
    delta_v_ = single([0;0;0]);
    v_reset_counter_ = 0;
end
resetNum = 0;
resetTotalNum = length(ModelReset_time);
if ~isempty(ModelReset_time)
    for i=1:resetTotalNum
        if resetTotalNum < 1.5
            if timestamp >= ModelReset_time(1)
                resetNum = 1;
                break;
            end
        else
            if i>=resetTotalNum
                if timestamp >= ModelReset_time(i)
                    resetNum = i;
                    break;
                end
            else
                if timestamp >= ModelReset_time(i) && timestamp < ModelReset_time(i+1)
                    resetNum = i;
                    break;
                end
            end
        end
    end
    if resetNum >0
        %         delta_p = p - p_last;
        if v_reset_counter_ ~= resetNum
            delta_v_ = v - v_last;
            v_reset_counter_ = resetNum;
        end
        v_last = v;
%         delta_xy_ = delta_p(1:2);
%         delta_z_ = delta_p(3);
%         delta_vxy_= delta_v(1:2);
%         delta_vz_ = delta_v(3);
%         delta_heading_ = heading - heading_last;
%         delta_q = quatmultiply(q(:)',quatconj(q_last(:)'));
%         delta_q_reset_ = delta_q(:);
        delta_xy = single(ModelReset_Pos(resetNum,1:2)');
        delta_z = single(ModelReset_Pos(resetNum,3));
        delta_heading = single(ModelReset_Euler(resetNum,3));
        delta_q = eul2quat([ModelReset_Euler(resetNum,3) ModelReset_Euler(resetNum,2) ModelReset_Euler(resetNum,1)],'ZYX');
        delta_q_reset = single(delta_q(:));
    else
        delta_xy = single([0;0]);
        delta_z = single(0);
%         delta_vxy = single([0;0]);
%         delta_vz = single(0);
        delta_heading = single(0);
        delta_q_reset = single([1;0;0;0]);
        v_last = v;
    end

else
    delta_xy = single([0;0]);
    delta_z = single(0);
%     delta_vxy = single([0;0]);
%     delta_vz = single(0);
    delta_heading = single(0);
    delta_q_reset = single([1;0;0;0]);
    v_last = v;
end
delta_vxy= delta_v_(1:2);
delta_vz = delta_v_(3);
xy_reset_counter = resetNum;
z_reset_counter = resetNum;
vxy_reset_counter = resetNum;
vz_reset_counter = resetNum;
heading_reset_counter = resetNum;
quat_reset_counter = resetNum;

== matlab function LW_ctrl_241029_1/states_update/vehicle_local_position/Sim/DisturbanceEstimator ==
  data: Va input; qm input single; omegam input single; T input single; ModelParam_uavJ parameter; ModelParam_motorJm parameter; ModelParam_rotorEta parameter; ModelParam_rotordx parameter; ModelParam_rotordy parameter; ModelParam_rotorCm parameter; ModelParam_rotorCt parameter; qk_ output; omegak_ output; d_hat output single size=[3,1]; LW_TEST_WNXY parameter; LW_TEST_WNZ parameter; LW_TEST_LAMXY parameter; LW_TEST_LAMZ parameter; LW_TEST_SIGXY parameter; LW_TEST_SIGZ parameter; ModelParam_LBb parameter; ModelParam_LBc parameter; ModelParam_LBS parameter; LW_ANGLE parameter; ModelParam_LBRho parameter; LW_USE_SER parameter; LW_LBCL_D parameter; LW_LBCM_D parameter; ModelParam_LBCn_d parameter; LW_TEST_TDT parameter; quat_reset_counter input; delta_q_reset input; dt input single
function [qk_, omegak_, d_hat] = DisturbanceEstimator(Va, qm, omegam, T,...
    ModelParam_uavJ,ModelParam_motorJm, ModelParam_rotorEta, ModelParam_rotordx, ModelParam_rotordy, ModelParam_rotorCm, ModelParam_rotorCt,...
    LW_TEST_WNXY, LW_TEST_WNZ,LW_TEST_LAMXY, LW_TEST_LAMZ, LW_TEST_SIGXY, LW_TEST_SIGZ, ModelParam_LBb, ModelParam_LBc, ModelParam_LBS, LW_ANGLE, ...
    ModelParam_LBRho, LW_USE_SER, LW_LBCL_D, LW_LBCM_D, ModelParam_LBCn_d, LW_TEST_TDT, quat_reset_counter, delta_q_reset, dt)

persistent tau_qk tau_omegak tau_z3
persistent  quat_reset_counter_
if isempty(quat_reset_counter_)
    quat_reset_counter_ = quat_reset_counter;
end

if isInfNan(qm)
    qm = single([1;0;0;0]);
else
    %qm = qm/(sqrt(qm'*qm));
    %qm = quatnormalize(qm');
    qm = qm(:);
end
if isInfNan(omegam)
    omegam = single([0;0;0]);
else
    omegam = omegam(:);
end
if isInfNan(T)
    T = single([0;0;0;0;0;0]);
else
    T = T(:);
end
if dt < 0.001
    dt = single(0.001);
elseif dt > 0.02
    dt = single(0.02);
end

if isempty(tau_qk)
    if notInfNan(qm)
        tau_qk = qm;
    else
        tau_qk = single([1;0;0;0]);
    end
end
if isInfNan(tau_qk)
    if notInfNan(qm)
        tau_qk = qm;
    else
        tau_qk = single([1;0;0;0]);
    end
end
if isempty(tau_omegak)
    if notInfNan(omegam)
        tau_omegak = omegam;
    else
        tau_omegak = single([0;0;0]);
    end
end
if isInfNan(tau_omegak)
    if notInfNan(omegam)
        tau_omegak = omegam;
    else
        tau_omegak = single([0;0;0]);
    end
end
if isempty(tau_z3)
    tau_z3 = single([0;0;0]);
end
if isInfNan(tau_z3)
    tau_z3 = single([0;0;0]);
end



%结构参数
rotorEta = single(ModelParam_rotorEta);
rotordx = single(ModelParam_rotordx);
rotordy = single(ModelParam_rotordy);
LBb = single(ModelParam_LBb);
LBc = single(ModelParam_LBc);
LBS = single(ModelParam_LBS);
kappa = single(LW_ANGLE*pi/180);
Rho = single(ModelParam_LBRho);
%动力系统参数
rotorCm = single(ModelParam_rotorCm);
rotorCt = single(ModelParam_rotorCt);
km_f = rotorCm/rotorCt;
Cl_d = single(LW_LBCL_D);
Cm_d = single(LW_LBCM_D);
Cn_d = single(ModelParam_LBCn_d);
%
Va_ = max(Va,0.1);
if LW_USE_SER > 0.5
    Q = 0.5*Rho*Va_^2*LBS;
else
    Q = single(0);
end
%滤波器参数
L = eye(3,2,"single");
wn = [LW_TEST_WNXY;LW_TEST_WNXY;LW_TEST_WNZ];%rad/s
sigma = [LW_TEST_SIGXY;LW_TEST_SIGXY;LW_TEST_SIGZ];
L(:,1) = wn.^2;
L(:,2) = 2*sigma.*wn;
lamda = single([LW_TEST_LAMXY;LW_TEST_LAMXY;LW_TEST_LAMZ]);
%滤波器结构
%reset处理
if quat_reset_counter_ ~= quat_reset_counter
    tau_q = quatmultiply(delta_q_reset(:)',tau_qk');
    tau_qk = tau_q';
    quat_reset_counter_ = quat_reset_counter;
end
q_err = quatmultiply(quatconj(tau_qk'), qm');
q_err = quatnormalize(q_err);
eta = constrain(q_err(1), single(-1), single(1));
epsilon = q_err(2 : 4);
theta = 2 * acos(eta);
theta = wrap_pi(theta);
if abs(theta) < 0.0873 % 5*pi/180
    Xi_e = sign(eta) * 2 * epsilon;
else
    Xi_e = sign(eta) / sin(theta / 2) * theta * epsilon;
end
e_q = Xi_e(:);
e_omega = omegam - tau_omegak;

%inv_uavJ = eye(3,3)/ModelParam_uavJ;
inv_uavJ = eye(3);
for ii = 1:3
    inv_uavJ(ii,ii) = 1/(ModelParam_uavJ(ii,ii));
end
%le = l1*eq+l2*ew
Le = L(:,1).*e_q + L(:,2).*e_omega;
K1 = km_f;
coseta = cos(rotorEta);
K2 = rotordy*coseta;
dxcoseta = rotordx*coseta;
%估计螺旋桨推力，根据混控器输出滤波得到
T = LowPass(T, LW_TEST_TDT);
B = [-K2       -K2        K2       K2      -Q*LBb*Cl_d*cos(kappa) Q*LBb*Cl_d*cos(kappa);
     dxcoseta  -dxcoseta dxcoseta -dxcoseta Q*LBc*Cm_d Q*LBc*Cm_d;
     K1        -K1       -K1      K1      Q*LBb*Cl_d*sin(kappa) -Q*LBb*Cl_d*sin(kappa)];
z3_ = tau_z3 + lamda.*Le*dt;
if LW_USE_SER > 0.5
    Fr = B*T;
else
    Fr = B(:,1:4)*T(1:4);
end

omegak_ = tau_omegak +(Le + z3_ + inv_uavJ*Fr- inv_uavJ*(cross(omegam,ModelParam_uavJ*omegam)))*dt;
delta_theta = [0 -omegak_(1) -omegak_(2) -omegak_(3);
               omegak_(1) 0 omegak_(3) -omegak_(2);
               omegak_(2) -omegak_(3) 0 omegak_(1);
               omegak_(3) omegak_(2) -omegak_(1) 0]*dt;
qk_ = (eye(4) + delta_theta/2)*tau_qk;
qk_ = qk_/(sqrt(qk_'*qk_));
d_hat = ModelParam_uavJ*(Le + z3_);

if notInfNan(z3_) && notInfNan(omegak_) && notInfNan(qk_)
    tau_z3 = z3_;
    tau_omegak = omegak_;
    tau_qk = qk_;
else
    tau_z3 = single([0;0;0]);
    tau_omegak = omegam;
    tau_qk = qm;
end

end

function d_est = LowPass(d_est,DT)
% DT = dt/(dt + Ts)
% 其中dt是采样周期，Ts是低通滤波器的时间常数
% 截止频率f = 1/Ts/2pi Hz
% 如 dt=0.004, f=30Hz , LW_TEST_DT=0.43
persistent d_est_last
if isempty(d_est_last)
    d_est_last = d_est;
end
if isInfNan(d_est_last)
    d_est_last = zeros(size(d_est),'single');
end
d_est = d_est_last + DT*(d_est - d_est_last);
d_est_last = d_est;
end

== matlab function LW_ctrl_241029_1/states_update/vehicle_local_position/HIL&FLY V1.13.3/nan_inf0 ==
  data: u input; y output
function y = fcn(u)

for i = 1:length(u)
    if isnan(u(i)) || isinf(u(i))
        u(i) = single(0);
    end
end
y = u(:);

== matlab function LW_ctrl_241029_1/states_update/vehicle_local_position/HIL&FLY V1.13.3/nan_inf1 ==
  data: u input; y output
function y = fcn(u)

for i = 1:length(u)
    if isnan(u(i)) || isinf(u(i))
        u(i) = single(0);
    end
end
y = u;

== matlab function LW_ctrl_241029_1/states_update/vehicle_local_position/Sim/nan_inf0 ==
  data: u input; y output
function y = fcn(u)

for i = 1:length(u)
    if isnan(u(i)) || isinf(u(i))
        u(i) = single(0);
    end
end
y = u;
